simulink library "CampusEnergyModeling"  (Simulink 8.1)
settings: Solver=ode45  StartTime=0.0  StopTime=10.0  RelTol=1e-3
undefined symbols (not defined in the file): a, b, c, j, look_Pin, look_Pout, magnitude
libraries: powerlib x6, simulink x3
(part 1 of 2)
settings Model: Creator=sfrank1  LastModifiedBy=sfrank1

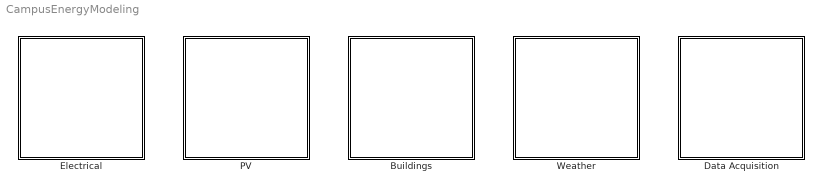
== system CampusEnergyModeling ==
  Buildings : Subsystem  Tag=Weather  Description=Contains blocks for acquiring and manipulating weather data.
      mask Display: disp('Buildings')
  Data Acquisition : Subsystem  Tag=Weather  Description=Contains blocks for acquiring and manipulating weather data.
      mask Display: disp('Data\nAcquisition')
  Electrical : Subsystem  Tag=Weather  Description=Contains blocks for acquiring and manipulating weather data.
      mask Display: disp('Electrical')
  PV : Subsystem  Tag=Weather  Description=Contains blocks for acquiring and manipulating weather data.
      mask Display: disp('PV')
  Weather : Subsystem  Tag=Weather  Description=Contains blocks for acquiring and manipulating weather data.
      mask Display: disp('Weather')

== system CampusEnergyModeling/Buildings ==
  EnergyPlus : M-S-Function  FunctionName=mlep_sfun  Parameters=work_dir, rel_path, fname, weather_profile, time_step, nout, timeout, eplus_path, bcvtb_dir, port, host  mask(EnergyPlus Cosimulation){work_dir=, rel_path=on, fname=idf_file, weather_profile=USA_IL_Chicago-OHare.Intl.AP.725300_TMY3, time_step=900, nout=2, timeout=10, mlep_defaults=on, eplus_path=, bcvtb_dir=, port=0, host=}
      mask prompts: work_dir "MLE+ working directory (empty = current directory)"; rel_path "Relative path"; fname "IDF file name"; weather_profile "EnergyPlus weather profile"; time_step "Time step (s)"; nout "Number of real outputs"; timeout "Communication timeout (s)"; mlep_defaults "Use default MLE+ settings"; eplus_path "EnergyPlus executable path (empty = default)"; bcvtb_dir "BCVTB directory (empty = default)"; port "Socket port (0 = auto)"; host "Socket host (empty = localhost)"
      mask help: This block implements cosimulation with EnergyPlus by allowing Simulink to exchange input and output data with it. Currently, EnergyPlus only supports real data.
      mask Help:
      | Simulate a building model using EnergyPlus
      | 
      | <h2>Description</h2>
      | This block implements <a href="http://apps1.eere.energy.gov/buildings/energyplus/">EnergyPlus</a> cosimulation by allowing Simulink to exchange input and output data with EnergyPlus at each time step.
      | 
      | When a simulation starts, this block starts EnergyPlus in parallel. During simulation, EnergyPlus exchanges data with Simulink using the <a href="http://simulationresearch.lbl.gov/bcvtb">Building Controls Virtual Test Bed</a> (BCVTB) interface via <a href="http://mlab.seas.upenn.edu/mlep/">MLE+</a>.
      | 
      | Detailed information about the interface is available in the MLE+ manual.
      | 
      | <h2>Requirements</h2>
      | Requires <a href="http://apps1.eere.energy.gov/buildings/energyplus/">EnergyPlus</a> and <a href="http://mlab.seas.upenn.edu/mlep/">MLE+</a>. In addition, requires a properly configured EnergyPlus model file (IDF) and BCVTB configuration file; see Comments.
      | 
      | <h2>Input</h2>
      | Block input <b>input</b> is a real-valued vector of EnergyPlus inputs corresponding to the inputs listed in the BCVTB config file <code>variables.cfg</code> (in order).
      | 
      | <h2>Output</h2>
      | The block outputs are, in order:
      | <dl>
      |   <dt><b>flag</b></dt><dd>Status flag for EnergyPlus: 0 if OK, non-zero for error</dd>
      |   <dt><b>time</b></dt><dd>Current simulation time of EnergyPlus (s)</dd>
      |   <dt><b>output</b></dt><dd>Real-valued vector of EnergyPlus outputs corresponding to the outputs listed in the BCVTB config file <code>variables.cfg</code> (in order).</dd>
      | </dl>
      | 
      | <h2>Parameters</h2>
      | The block mask provides inputs for all required MLE+ configuration parameters. The mask includes two tabs. The <i>Model</i> tab provides information about the EnergyPlus model to run, and the <i>MLE+</i> provides inputs for MLE+ settings.
      | 
      | String inputs in the block mask, such as paths and file names, are not evaluated prior to passing to MLE+. Therefore, MATLAB expressions which evaluate to strings (for example, <code>[pwd '/somedir']</code>) may not be passed directly. Instead, use an initialization script to evaluate these expressions and store the evaluated strings in the block mask prior to running the simulation.
      | 
      | <h3>Model Tab</h3>
      | The <i>Model</i> tab provides inputs for the following parameters:
      | <dl>
      |   <dt><b>MLE+ working directory</b></dt>
      |     <dd>The MLE+ and EnergyPlus working directory. <i>EnergyPlus will read from and write to this directory.</i></dd>
      |   <dt><b>Relative path</b></dt>
      |     <dd>Check this box if <b>MLE+ working directory</b> is specified relative to the current MATLAB working directory. <i>Otherwise, the block will treat <b>MLE+ working directory</b> as an absolute path.</i></dd>
      |   <dt><b>IDF file name</b></dt>
      |     <dd>The EnergyPlus model file (IDF), with or without the <code>.idf</code> extension. <i>This file must be included in the <b>MLE+ working directory</b>. Do not specify an absolute path for this file!</i></dd>
      |   <dt><b>EnergyPlus weather profile</b></dt>
      |     <dd>The EnergyPlus weather file (EPW), with or without the <code>.epw</code> extension. <i>A matching weather file must be included in your EnergyPlus installation's <code>WeatherData</code> directory.</i></dd>
      |   <dt><b>Time Step</b></dt>
      |     <dd>The EnergyPlus time step (s). <i>This need not be the same as the Simulink time step.</i></dd>
      |   <dt><b>Number of Real Outputs</b></dt>
      |     <dd>The number of real outputs from EnergyPlus. <i>This number must match the number of output variables in <code>variables.cfg</code>.</i></dd>
      | </dl>
      | 
      | <h3>MLE+ Tab</h3>
      | The <i>MLE+</i> tab provides inputs for the following parameters:
      | <dl>
      |   <dt><b>Communication timeout</b></dt>
      |     <dd>Time delay (s) before communication between MLE+ and EnergyPlus times out.</dd>
      |   <dt><b>Use default MLE+ settings</b></dt>
      |     <dd>Uncheck this box to gain access to the remaining settings in the <i>MLE+</i> tab.</dd>
      |   <dt><b>EnergyPlus executable path</b></dt>
      |     <dd>The full path to the EnergyPlus executable (e.g. <code>C:\EnergyPlusV8-1-0\RunEPlus.bat</code>); leave blank to use default MLE+ setting.</dd>
      |   <dt><b>BCVTB directory</b></dt>
      |     <dd>The full path to the directory where the BCVTB library resides; leave blank to use default MLE+ setting.</dd>
      |   <dt><b>Socket port</b></dt>
      |     <dd>The port to use for communication with EnergyPlus; enter <code>0</code> to allow MLE+ to automatically select a port.</dd>
      |   <dt><b>Socket host</b></dt>
      |     <dd>The IP address of the host machine where EnergyPlus runs; leave blank to use localhost (the local computer).</dd>
      | </dl>
      | 
      | <h2>Comments</h2>
      | <ol>
      |   <li>For fixed time step simulation in Simulink, the EnergyPlus time step must be an exact multiple of the Simulink time step.</li>
      |   <li>Summary of requirements for EnergyPlus model file (<code>*.idf</code>):
      |     <ol type="a">
      | 	  <li>The EnergyPlus time step specified in the file must match the value specified in the block mask.</li>
      | 	  <li>The start date and time in EnergyPlus must correspond to the start time of the Simulink simulation (usually <i>t</i> = 0 s).</li>
      | 	  <li>The <i>ExternalInterface</i> object must be defined and assigned the name  <code>PtolemyServer</code>.</li>
      | 	  <li>The file must include <i>ExternalInterface</i> definitions all inputs specified in the BCVTB config file, and the names must match.</li>
      | 	  <li>The file must include <i>Output</i> definitions all outputs specified in the BCVTB config file, and the names must match.</li>
      | 	</ol>
      |   </li>
      |   <li>Summary of requirements for BCVTB config file (<code>variables.cfg</code>):
      |     <ol type="a">
      | 	  <li>The file be located in the MLE+ working directory specified in the block mask.</li>
      | 	  <li>Number of output variables must match the value specified in the block mask.</li>
      | 	  <li>Order of input variables must match the order of elements in the input vector in Simulink.</li>
      | 	  <li>Order of output variables must match the order of elements in the output vector in Simulink.</li>
      | 	</ol>
      |   <li>For more details regarding the implementation of MLE+, the meaning of the parameters, and creating the BCVTB configuration file, see the MLE+ <a href="http://mlab.seas.upenn.edu/mlep/">documentation</a>.</li>
      | </ol>
      | 
      | <h2>References</h2>
      | <ol>
      |   <li>W. Bernal, M. Behl, T. X. Nghiem, and R. Mangharam, "MLE+: A Tool for Integrated Design and Deployment of Energy Efficient Building Controls," 4th ACM Workshop On Embedded Sensing Systems For Energy-Efficiency In Buildings, (BuildSys '12), Toronto, Canada, 2012. Available: <a href="http://repository.upenn.edu/mlab_papers/51/">http://repository.upenn.edu/mlab_papers/51/</a></li>
      | </ol>
      mask Callback mlep_defaults: EnergyPlus_cb(gcb, 'mlep_config');
      mask Display:
      | image(imread('building.png'))
      | disp('EnergyPlus\nCosimulation');
      | 
      | % Inputs
      | port_label('input', 1, 'input');
      | 
      | % Outputs
      | port_label('output', 1, 'flag');
      | port_label('output', 2, 'time');
      | port_label('output', 3, 'output');

== system CampusEnergyModeling/Data Acquisition ==

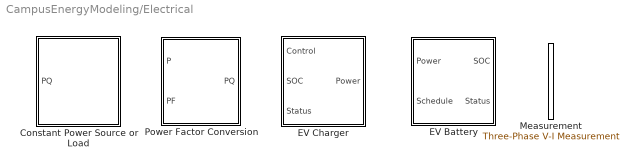
== system CampusEnergyModeling/Electrical ==
  Constant Power Source or Load : Subsystem  mask(Constant Power Source/Load){Conven=source, PNom=5000, QNom=2000, VNom=480, fNom=60, VLow=0.7}
      mask prompts: Conven "Electrical convention"; PNom "Nominal three-phase real power (W)"; QNom "Nominal three-phase reactive power (VAR)"; VNom "Nominal line-to-line voltage (VRMS)"; fNom "Nominal frequency (Hz)"; VLow "Lower voltage limit (pu)"
      mask help: Implements a controllable three-phase, constant power source or load, where VI* = P + jQ (in per-unit).
      mask init:
      | % Call initialization to calculate block variables
      | InputGain = ...
      |     ConstantPowerSourceLoad_cb(gcb, 'init', ...
      |     Conven, PNom, QNom, VNom, fNom, VLow);
      mask Help:
      | Supply or consume constant three-phase power
      | 
      | <h2>Description</h2>
      | This block implements a controllable three-phase, constant power source or load in SimPowerSystems (phasor mode). The load characteristic is given by
      | <blockquote>
      |   <i>P</i> + <i>jQ</i> = sqrt(3) · <i>VI</i><sup>*</sup>,
      | </blockquote>
      | in which
      | <blockquote>
      |   <i>V</i> = Positive sequence line-to-line voltage (V)<br/>
      |   <i>I</i> = Positive sequence phase current (A)<br/>
      |   <i>P</i> = Positive sequence real power (from PQ input)<br/>
      |   <i>Q</i> = Positive sequence reactive power (from PQ input)
      | </blockquote>
      | 
      | The block supplies <i>P</i> + <i>jQ</i> if the source convention is specified and consumes <i>P</i> + <i>jQ</i> if the load convention is specified.
      | 
      | <h2>Requirements</h2>
      | Requires SimPowerSystems.
      | 
      | <h2>Input</h2>
      | Input <b>PQ</b> is a two dimensional vector [<i>P</i>, <i>Q</i>] specifying the real and reactive power consumption (for a load) or generation (for a source).
      | 
      | <h2>Physical Ports</h2>
      | <p>The block has a three-phase, four-wire physical representation in SimPowerSystems. The physical ports are:
      | <dl>
      |   <dt><b>A</b></dt><dd>Phase A electrical connection</dd>
      |   <dt><b>B</b></dt><dd>Phase B electrical connection</dd>
      |   <dt><b>C</b></dt><dd>Phase C electrical connection</dd>
      |   <dt><b>N</b></dt><dd>Neutral electrical connection</dd>
      | </dl>
      | </p>
      | 
      | <h2>Parameters</h2>
      | <dl>
      |   <dt><b>Electrical convention</b></dt>
      |     <dd>Specifies whether the block is a source or a load</dd>
      |   <dt><b>Nominal three-phase real power</b></dt>
      |     <dd>The nominal real power production (consumption) for the source (load), in W</dd>
      |   <dt><b>Nominal three-phase reactive power</b></dt>
      |     <dd>The nominal reactive power production (consumption) for the source (load), in W</dd>
      |   <dt><b>Nominal line-to-line voltage</b></dt>
      |     <dd>The nominal line-to-line voltage, in V</dd>
      |   <dt><b>Nominal frequency</b></dt>
      |     <dd>The nominal frequency of the device, in Hz</dd>
      |   <dt><b>Lower voltage limit</b></dt>
      |     <dd>The voltage below which the block converts to a constant current device; see Comments</dd>
      | </dl>
      | 
      | <h2>Comments</h2>
      | <ol>
      |   <li>This block is compatible with SimPowerSystems' <b>phasor simulation mode only.</b></li>
      |   <li>The nominal input fields in the mask are used to initialize the block parameters. If the nominal values are close to the actual values during simulation, then the block will converge more rapidly.</li>
      |   <li>If the positive sequence voltage falls below the per-unit lower voltage limit (on the base specified by the nominal line-to-line voltage), then the block will behave as a constant current source rather than a constant power source, with the current magnitude capped at the level required to supply full power at the lower voltage limit. This feature avoids current runaway that would otherwise occur during voltage collapes. By default, the lower voltage limit is <i>V</i> = 0.7 pu.
      | </ol>
      mask TypeOptions Conven: source | load
  EV Battery : Subsystem  mask(Electric Vehicle Battery){capacity=24000, initSOC=0.3}
      mask prompts: capacity "Battery capacity (Wh)"; initSOC "Initial state of charge (fraction)"
      mask help: Implements an idealized (lossless) model for an electric vehicle (EV) battery.
      mask Help:
      | Models a lossless electric vehicle battery
      | 
      | <h2>Description</h2>
      | This block models an idealized (lossless) electric vehicle (EV) battery. The battery is modeled using a simple integrator on the input power, capped at 100% state of charge (SOC). Battery SOC resets to a specified initial value whenever the EV reconnects to the charging station (whenever the <b>Schedule</b> input transitions from 0 to 1).
      | 
      | <h2>Input</h2>
      | <dl>
      |   <dt><b>Power</b></dt>
      |     <dd>Battery charging power (W)</dd>
      |   <dt><b>Schedule</b></dt>
      |     <dd>EV schedule:
      |         <ul>
      |           <li>1 (or any other positive number) if the EV is connected to the charging station,</li>
      |           <li>0 otherwise.</li>
      |         </ul>
      |     </dd>
      |     </dl>
      | </dl>
      | 
      | <h2>Output</h2>
      | <dl>
      |   <dt><b>SOC</b></dt>
      |     <dd>EV battery current state of charge (fraction); compatible with the <b>SOC</b> input of the <i>EV Charger</i> block</dd>
      |   <dt><b>Status</b></dt><dd>EV status:
      |     <ul>
      |       <li>&minus;1 for not present,</li>
      |       <li>0 for present and accepting charge,</li>
      |       <li>1 for present but battery full;</li>
      |     </ul>
      |     compatible with the <b>Status</b> input of the <i>EV Charger</i> block</dd>
      | </dl>
      | 
      | <h2>Parameters</h2>
      | <dl>
      |   <dt><b>Battery capacity</b></dt>
      |     <dd>EV battery storage capacity (Wh)</dd>
      |   <dt><b>Initial state of charge</b></dt>
      |     <dd>Initial battery SOC when the battery first reconnects to the charging station (fraction)</dd>
      | </dl>
  EV Charger : Subsystem  mask(Electric Vehicle Charging Station){rating=6240, capacity=24000, maxresponse=1000, ramp=1000}
      mask prompts: rating "Charger rating (W)"; capacity "Connected EV battery capacity (Wh)"; maxresponse "Desired +/- regulatory response capability (W)"; ramp "Maximum ramp rate (W/s)"
      mask help: Implements a simple model for an electric vehicle charging station. Accepts connections for the EV state of charge and status as well as an external control signal requesting a regulatory deviation from the current charging setpoint. Outputs a charging power.
      mask Help:
      | Models an electric vehicle charging station
      | 
      | <h2>Description</h2>
      | This block models an idealized electric vehicle (EV) charging station. It is an approximation of how actual EV charging stations operate (to be updated in a later release of the library). The charger uses a preset charging power profile based on the EV battery state of charge (SOC). As the SOC approaches 100%, the charger tapers the charge rate to zero. In addition, the charger monitors the connection status of the EV and sets charging power to zero if the EV is disconnected or has a full battery.
      | 
      | The block has a <b>Control</b> signal which requests regulatory control of the EV charging load as a deviation from the current charging setpoint. This allows the EV charger to participate in demand response or regulation of distributed generation (such as smoothing output from a photovoltaic array). The charger attempts to maintain the active response capability specified in the block mask by operating at less than maximum charging capacity. It can then respond to the control signal within its present charging limits. See Comments for details.
      | 
      | <h2>Input</h2>
      | <dl>
      |   <dt><b>Control</b></dt>
      |     <dd>Signal requesting regulatory control of charging power (&plusmn; deviation from charging setpoint) (W)</dd>
      |   <dt><b>SOC</b></dt>
      |     <dd>EV battery current state of charge (fraction); compatible with the <b>SOC</b> output of the <i>EV Battery</i> block</dd>
      |   <dt><b>Status</b></dt>
      |     <dd>EV status:
      |     <ul>
      |       <li>&minus;1 for not present,</li>
      |       <li>0 for present and accepting charge,</li>
      |       <li>1 for present but battery full;</li>
      |     </ul>
      |     compatible with the <b>Status</b> output of the <i>EV Battery</i> block</dd>
      | </dl>
      | 
      | <h2>Output</h2>
      | Output <b>Power</b> is the charger power output (W).
      | 
      | <h2>Parameters</h2>
      | <dl>
      |   <dt><b>Charger rating</b></dt>
      |     <dd>The charger maximum power rating (W)</dd>
      |   <dt><b>Connected EV battery capacity</b></dt>
      |     <dd>The total energy storage capacity of the connected EV battery (Wh)</dd>
      |   <dt><b>Desired +/- regulatory response capability</b></dt>
      |     <dd>The target control response capability (W) for the charger</dd>
      |   <dt><b>Maximum ramp rate</b></dt>
      |     <dd>Maximum charging ramp rate (&plusmn; rate of change in charging power) (W/s)</dd>
      | </dl>
      | 
      | <h2>Comments</h2>
      | Internally, the block sets a maximum charge rate based on the EV battery capacity and current SOC. The charging setpoint is the maximum rate less any requested regulatory response capability. The actual charging power is equal to this setpoint plus the effect of the control signal.
      | 
      | The ability of the charger to respond to the requested control action is limited by four factors:
      | <ol>
      |   <li>The output power cannot exceed the specified charger power rating.</li>
      |   <li>The output power cannot exceed the maximum charge rate defined by the battery charging profile.</li>
      |   <li>The output power cannot be less than zero. (The battery cannot be discharged to the grid.)</li>
      |   <li>The output power cannot change at a rate greater than the specified maximum ramp rate.</li>
      | </ol>
      | 
      | <i>Example:</i> If, given the current battery SOC, the charging profile for the EV battery specifies 5000 W and the requested regulatory response capability is &plusmn;1000 W, then the EV charger will charge at a setpoint of 4000 W &plusmn; the requested control action, within the limits of the charger. If the requested control action is &minus;500 W, then the EV charger will reduce output to 4000 &minus; 500 = 3500 W.
  Measurement : powerlib/Measurements/Three-Phase V-I Measurement  VoltageMeasurement=phase-to-ground  SetLabelV=on  LabelV=Vabc_1  Vpu=off  VpuLL=off  CurrentMeasurement=yes  SetLabelI=on  LabelI=Iabc_1  Ipu=off  Pbase=1e6  Vbase=25e3  OutputType=Complex  PhasorSimulation=on  PSBequivalent=0
  Power Factor Conversion : Subsystem  mask(Power Factor Conversion){pfType=Lagging}
      mask prompts: pfType "Type of power factor"
      mask help: Converts a real input power and power factor to a vector of real and reactive power.
      mask init:
      | % Set multiplier for Q based on load type
      | if pfType == 1
      |     % Leading
      |     leadlag = -1;
      | else
      |     % Lagging
      |     leadlag = 1;
      | end
      mask Help:
      | Convert from real power and power factor to real and reactive power
      | 
      | <h2>Description</h2>
      | 
      | Given a real input power and power factor, this block computes a vector of real and reactive power (compatible with the <i>Constant Power Source/Load</i> block). Reactive power <i>Q</i> in output vector [<i>P</i>, <i>Q</i>] is given by
      | <blockquote>
      |   <i>Q</i> = &plusmn;<i>P</i> · sqrt( 1 + 1 / PF&sup2; ),
      | </blockquote>
      | with the sign determined by whether the power factor is assumed to be lagging (+) or leading (&minus;) (selectable in the block mask).
      | 
      | <h2>Input</h2>
      | Input <b>P</b> is the real power and input <b>PF</b> is the power factor.
      | 
      | <h2>Output</h2>
      | Output <b>PQ</b> is a two dimensional vector [<i>P</i>, <i>Q</i>] of the computed real and reactive power.
      | 
      | <h2>Parameters</h2>
      | The <b>type of power factor</b> parameter is a drop-down list which specifies whether the power factor is leading or lagging.
      mask TypeOptions pfType: Leading | Lagging

== system CampusEnergyModeling/PV ==
  Generic Inverter : Subsystem  mask(Generic Inverter){model_type=Fixed Efficiency, fixed_eff=0.95, alpha=1, beta=0.01, gamma=0.001, lookup_pair=Input Power + Output Power, lookup_in=[0, 10, 25, 50, 75, 100], lookup_out=[0, 9, 24, 49, 73, 97], lookup_eff=[0.10, 0.80, 0.87, 0.93, 0.90, 0.88], standby=0}
      mask prompts: model_type "Inverter model"; fixed_eff "Efficiency"; alpha "Constant loss coefficient (W)"; beta "Linear loss coefficient (W/W)"; gamma "Quadratic loss coefficient (W/W²)"; lookup_pair "Specify..."; lookup_in "Input power (W)"; lookup_out "Output power (W)"; lookup_eff "Efficiency"; standby "Standby Loss (W)"
      mask help:
      | Implements the efficiency characteristic for a generic PV inverter using one of three models:
      | - Fixed efficiency
      | - Quadratic loss model
      | - Lookup table
      |
      | See the help for details for each of these models.
      mask init:
      | % Call initialization to calculate block variables
      | [a, b, c, look_Pin, look_Pout] = ...
      |     GenericInverter_cb(gcb, 'init', model_type, ...
      | 	fixed_eff, alpha, beta, gamma, ...
      |     lookup_pair, lookup_in, lookup_out, lookup_eff);
      mask Help:
      | Simulate the efficiency characteristic of a generic PV inverter
      | 
      | <h2>Description</h2>
      | The block simulates the efficiency characteristic of a generic photovoltaic (PV) inverter using one of three models:
      | <ul>
      |   <li>Fixed efficiency</li>
      |   <li>Quadratic loss model</li>
      |   <li>Lookup table</li>
      | </ul>
      | 
      | <h3>Fixed Efficiency Model</h3>
      | Under the fixed efficiency model, the inverter power output is a fixed fraction of the input: <i>P<sub>out</sub></i> = <i>&eta;</i><i>P<sub>in</sub></i>. Efficiency <i>&eta;</i> is a mask parameter.
      | 
      | <h3>Quadratic Loss Model</h3>
      | Under the quadratic loss model, inverter losses are a quadratic function of the inverter input power. The power relationship is <i>P<sub>out</sub></i> = <i>P<sub>in</sub></i> - ( <i>&alpha;</i> + <i>&beta;</i><i>P<sub>in</sub></i> + <i>&gamma;</i><i>P<sub>in</sub></i>²). <i>&alpha;</i>, <i>&beta;</i>, and <i>&gamma;</i> are the constant, linear, and quadratic loss coefficients, respectively, and are mask parameters.
      | 
      | <h3>Lookup Table</h3>
      | Inverter output power is computed as a function of the input power using interpolation from a preset lookup table.
      | 
      | <h2>Input</h2>
      | Block input <b>Pin</b> is the inverter input power.
      | 
      | <h2>Output</h2>
      | Block output <b>Pout</b> is the inverter output power.
      | 
      | <h2>Parameters</h2>
      | <b>Standby loss</b> (W) specifies the inverter power consumption when the array is dark. The remaining parameters available in the block mask depend on which <b>inverter model</b> is selected in the mask dialog.
      | 
      | <h3>Fixed Efficiency Model</h3>
      | Specify the fixed inverter <b>efficiency</b> <i>&eta;</i> as a fraction.
      | 
      | <h3>Quadratic Loss Model</h3>
      | Specify <i>&alpha;</i>, <i>&beta;</i>, and <i>&gamma;</i> in the inverter loss equation:
      | <dl>
      |   <dt><b>Constant loss coefficient</b></dt><dd>Specify the constant inverter loss <i>&alpha;</i> (W).</dd>
      |   <dt><b>Linear loss coefficient</b></dt><dd>Specify the linear inverter loss coefficient <i>&beta;</i> (W/W).</dd>
      |   <dt><b>Quadratic loss coefficient</b></dt><dd>Specify the quadratic inverter loss coefficient <i>&gamma;</i> W/W²).</dd>
      | </dl>
      | 
      | <h3>Lookup Table</h3>
      | Specify two of the following three vectors: <b>input power</b>, <b>output power</b>, and <b>efficiency</b>. Vector dimensions must match and efficiencies must be entered as fractions. The block automatically calculates the appropriate input-output power characteristic from the inputs provided according to the relationship <i>&eta;</i> = <i>P<sub>out</sub></i> / <i>P<sub>in</sub></i>.
      | 
      | <h2>Comments</h2>
      | <ol>
      |   <li>When the inverter input power drops too low to sustain a positive power output, the inverter drops into standby automatically, consuming the specified standby loss.</li>
      |   <li><i>Caution:</i> If using the lookup table model, do not include zeros in the efficiency vector. Otherwise, a divide by zero error may result.</li>
      | </ol>
      | 
      | <h2>References</h2>
      | For discussion of the quadratic inverter loss model, see section 3.4.4 of:
      | <ol>
      |   <li>S. Frank, "Optimal Design of Mixed AC-DC Distribution Systems for Commercial Buildings," Dissertation, Colorado School of Mines, Golden, CO, 2013. Available: <a href="http://gradworks.umi.com/3558161.pdf">http://gradworks.umi.com/3558161.pdf</a></li>
      | </ol>
      mask TypeOptions model_type: Fixed Efficiency | Quadratic | Lookup Table
      mask Callback model_type:
      | % Dynamic mask callback
      | GenericInverter_cb(gcb, 'model_type')
      mask TypeOptions lookup_pair: Input Power + Output Power | Input Power + Efficiency | Output Power + Efficiency
      mask Callback lookup_pair:
      | % Dynamic mask callback
      | GenericInverter_cb(gcb, 'lookup_pair')
  PV Smoothing : TransferFcn  Denominator=[tau 1]  mask(Photovoltaic Array Smoothing){sel=Array Size and Power Density, tc=15, area=33000, size=1e6, density=150, coverage=0.2}
      mask prompts: sel "Specify..."; tc "Time constant (s)"; area "Array area (m²)"; size "Array size (W)"; density "Panel nominal power density (W/m²)"; coverage "Panel ground coverage ratio (fraction)"
      mask help: Implements a low pass filter to model the smoothing effect of a utility-scale PV array.
      mask init:
      | % Call initialization to calculate block variables
      | tau = PVSmoothing_cb(gcb, 'init', ...
      |     sel, tc, area, size, density, coverage);
      mask Help:
      | Model the smoothing effect of a utility-scale PV array
      | 
      | <h2>Description</h2>
      | This block implements a low pass filter to model the smoothing effect of a utility-scale PV array per the empirical model presented in Marcos et al. (2011) (see References). The smoothing is done by a unity-gain low pass filter with transfer function
      | <blockquote>
      |   Output / Input = 1 / (<i>&tau;</i><i>s</i> + 1),
      | </blockquote>
      | in which time constant <i>&tau;</i> may either be defined directly or estimated from the array area. The empirical formula of Marcos et al. estimates <i>&tau;</i> as
      | <blockquote>
      |   <i>&tau;</i> = sqrt(<i>A</i>) / (2·&pi;·0.020)
      | </blockquote>
      | in which <i>A</i> is the physical array area in hectares (1 Ha = 10000 m&sup2;). Array area <i>A</i> may be specified directly or calculated from the array size, panel power density, and ground coverage ratio (defined as the fraction of ground area occupied by the actual PV panels).
      | 
      | <h2>Input</h2>
      | Block input <b>Pin</b> is the unsmoothed PV array power.
      | 
      | <h2>Output</h2>
      | Block output <b>Pout</b> is the smoothed PV array power.
      | 
      | <h2>Parameters</h2>
      | In the mask dialog, the user elects to specify the time constant, the array area, or the array size and power density.
      | 
      | <h3>Time Constant</h3>
      | Specify the <b>time constant</b> (s) for the low pass filter directly.
      | 
      | <h3>Array Area</h3>
      | Specify the <b>array area</b> (m&sup2;) and compute the time constant from the equation of Marcos et al. (2011).
      | 
      | <h3>Time Constant</h3>
      | Specify the <b>array size</b> (W), <b>nominal power density</b> (W/m&sup2;), and <b>ground coverage ratio</b> (fraction). From this, the block computes the approximate array area and the time constant from the equation of Marcos et al. (2011).
      | 
      | <h2>Comments</h2>
      | <ol>
      |   <li>This block includes a continuous time low pass filter. Therefore, the block may not be used with a discrete solver. Also, use caution when attempting to use this block within models with fixed time larger than the smoothing time constant; the Simulink solver may generate an error.</li>
      | </ol>
      | 
      | <h2>References</h2>
      | <ol>
      |   <li>J. Marcos et al., "From irradiance to output power fluctuations: the PV plant as a low pass filter", <i>Progress In Photovoltaics: Research And Applications</i>, 2011, 19, 505-510.</li>
      | </ol>
      mask TypeOptions sel: Time Constant | Array Area | Array Size and Power Density
      mask Callback sel: PVSmoothing_cb(gcb, 'dynamic_mask')
      mask Display: plot([1 2 3],[1 1 0])
  PVWatts Cosimulation : M-S-Function  FunctionName=pvwatts_sfun  Parameters=lat, lon, start_time, tz, time_step, system_size, derate, azimuth, tilt, track_mode, rotlim, t_ref, t_noct, gamma, i_ref, poa_cutin, init_tcell, init_poa, output_dc, output_celltemp, output_poa  mask(PVWatts Cosimulation){lat=39.74, lon=-105.18, start_time=2012-01-01 00:00:00, tz=-6, time_step=600, system_size=1000, derate=0.95, azimuth=180, tilt=39.74, use_lat_tilt=on, track_mode=Fixed, rotlim=45, use_cell_data=off, t_ref=25, t_noct=45, gamma=-0.5, i_ref=1000, poa_cutin=0, init_tcell=25, init_poa=0, output_dc=on, output_celltemp=on, output_poa=on}
      mask prompts: lat "Latitude"; lon "Longitude"; start_time "Initial date/time (yyyy-mm-dd HH:MM:SS)"; tz "Time zone (offset from UTC)"; time_step "Time step (s)"; system_size "Array nameplate capacity (W)"; derate "System derate factor (0-1)"; azimuth "Azimuth angle (N = 0°, E = 90°, S = 180°, W = 270°)"; tilt "Tilt angle"; use_lat_tilt "Use latitude tilt"; track_mode "Tracking mode"; rotlim "Tracker rotation limit (+/-)"; use_cell_data "Customize photovoltaic cell data"; t_ref "Reference cell temperature (°C)"; t_noct "Nominal operating cell temperature (°C)"; gamma "Maximum power temperature coefficient (%/°C)"; i_ref "Irradiance condition for cell rating (W/m²)"; poa_cutin "Minimum irradiance for operation (W/m²)"; init_tcell "Initial cell temperature (°C)"; init_poa "Initial plane of array irradiance (W/m²)"; output_dc "Output DC power (W)"; output_celltemp "Output cell temperature (°C)"; output_poa "Output plane of array irradiance (W/m²)"
      mask help:
      | This block implements cosimulation of a photovoltaic (PV) array using the PVWatts module of the SAM Simulation Code (SSC) SDK. Data entry is organized in four tabs:
      | 1. Time and Location: where the array is located and when the simulation occurs.
      | 2. Array: PV array nameplate rating and physical characteristics.
      | 3. Cell: Customized model parameters for the PV cells (optional).
      | 4. Simulation: Initial conditions and simulation options.
      |
      | See the block help for more information.
      mask init:
      | PVWatts_cb(gcb, 'redraw_mask');
      mask Help:
      | Simulate a photovoltaic array using PVWatts
      | 
      | <h2>Description</h2>
      | This block implements cosimulation of a photovoltaic (PV) array using the PVWatts (<code>pvwattsfunc</code>) module of the SAM Simulation Core (SSC) SDK. The cosimulation runs in SSC at the time step specified in the <i>Time and Location</i> parameter tab (which need not be identical to the Simulink time step).
      | 
      | Detailed documentation for the SSC SDK is available for download from the <a href="https://sam.nrel.gov/content/sam-simulation-core-sdk">SAM website<a/>; see References.
      | 
      | <h2>Requirements</h2>
      | Requires <a href="https://sam.nrel.gov/content/sam-simulation-core-sdk">SSC</a>.
      | 
      | <h2>Input</h2>
      | The block inputs accept weather data synced to the simulation time stamp:
      | <dl>
      |   <dt><b>Beam</b></dt><dd>Beam irradiance (W/m&sup2;)—Also known as "direct normal irradiance"</dd>
      |   <dt><b>Diffuse</b></dt><dd>Diffuse irradiance (W/m&sup2;)—Also known as "diffuse horizontal irradiance"</dd>
      |   <dt><b>Temp</b></dt><dd>Ambient temperature (&deg;C)</dd>
      |   <dt><b>Wind</b></dt><dd>Wind speed (m/s)</dd>
      | </dl>
      | 
      | <h2>Output</h2>
      | The block outputs are, in order:
      | <dl>
      |   <dt><b>DC Power</b></dt><dd>Array DC output power (W)</dd>
      |   <dt><b>Cell Temp</b></dt><dd>Array PV cell temperature (&deg;C)</dd>
      |   <dt><b>POA Irradiance</b></dt><dd>Plane of array incident irradiance (W/m&sup2;)</dd>
      | </dl>
      | 
      | Each output may be individually enabled or disabled on the <i>Simulation</i> tab. Enabling or disabling outputs will change the number of output ports on the block, possibly disrupting existing signal connections in Simulink.
      | 
      | <h2>Parameters</h2>
      | The block mask provides inputs for most (although not all) of the PV array model parameters available for PVWatts in SSC. The four input tabs in the block mask are
      | <ol>
      |   <li><i>Time and Location:</i> Specify where the array is located and when the simulation occurs. Includes fields for array <b>latitude</b> and <b>longitude</b>, the <b>initial date and time</b> (corresponding to simulation time <i>t</i> = 0), <b>time zone</b>, and PVWatts simulation <b>time step.</b></li>
      |   <li><i>Array:</i> Specify the PV array <b>nameplate capacity</b>, <b>derate factor</b>, and physical characteristics (<b>azimuth angle</b>, <b>tilt angle</b>, and <b>tracking mode</b>).</li>
      |   <li><i>Cell:</i> Allows customization of the photovoltaic cell data—<b>reference cell temperature</b>, <b>nominal operating cell temperature</b>, <b>maximum power temprature coefficient</b>, <b>irradiance condition</b> for cell rating, and <b>minimum irradiance</b> for cell operation.</li>
      |   <li><i>Simulation:</i> Specify the array initial conditions (<b>cell temperature</b> and <b>plane of array irradiance)</b> and select the desired block outputs.</li>
      | </ol>
      | 
      | For a detailed description of these parameters, see the SSC SDK documentation.
      | 
      | <h2>Comments</h2>
      | <ol>
      |   <li>The block is designed to model the DC operation of a PV array only. Therefore, no inverter efficiency mask parameter or AC power output are provided. To model inverter losses, apply an external inverter model to the DC power output, such as the Generic Inverter model available in the Campus Energy Modeling Simulink library.</li>
      |   <li><i>Caution:</i> Checking <b>Use latitude tilt</b> in the <i>Array</i> tab will discard the existing tilt angle and replace it with the absolute value of the latitude.</li>
      |   <li><i>Caution:</i> Unchecking <b>Customize photovoltaic cell data</b> in the <i>Cell</i> tab will discard any existing customizations in the PV cell data fields and replace them with default values.</li>
      |   <li>Additional description for the SSC module input and output variables may be obtained using the SSCdev application distributed with SSC SDK; see the SSC SDK documentation for usage instructions.</li>
      | </ol>
      | 
      | <h2>References</h2>
      | <ol>
      |   <li>National Renewable Energy Laboratory, "SAM Simulation Core SDK." Available: <a href="https://sam.nrel.gov/content/sam-simulation-core-sdk">https://sam.nrel.gov/content/sam-simulation-core-sdk</a></li>
      | </ol>
      mask Callback lat: PVWatts_cb(gcb, 'use_lat_tilt');
      mask Callback use_lat_tilt: PVWatts_cb(gcb, 'use_lat_tilt');
      mask TypeOptions track_mode: Fixed | 1-Axis | 2-Axis | Azimuth Axis
      mask Callback track_mode: PVWatts_cb(gcb, 'track_mode');
      mask Callback use_cell_data: PVWatts_cb(gcb, 'use_cell_data');
      mask Display:
      | % This mask display is automatically generated by PVWatts_cb()
      | image('pvwatts_light.png')
      | disp('PVWatts\nCosimulation')
      | 
      | % Label input ports
      | port_label('input', 1, 'Beam'); % Beam irradiance (W/m^2)
      | port_label('input', 2, 'Diffuse'); % Diffuse irradiance (W/m^2)
      | port_label('input', 3, 'Temp'); % Ambient temperature (deg C)
      | port_label('input', 4, 'Wind'); % Wind speed (m/s)
      | 
      | % Label output ports
      | port_label('output', 1, 'DC Power'); % DC output power (W)
      | port_label('output', 2, 'Cell Temp'); % Cell temperature (deg C)
      | port_label('output', 3, 'POA Irradiance'); % % Point of array irradiance

== system CampusEnergyModeling/Weather ==
  Weather Data : Subsystem  mask(Weather Data From File){fname=TMY3.mat, initbus=off}
      mask prompts: fname "Weather file"; initbus "Create Simulink bus definition automatically"
      mask help:
      | Reads weather data from the specified binary file and outputs it as a Simulink bus signal.
      |
      | The utility function convertTMY3() to creates a .MAT file compatible with this block. Use of this block requires that a Simulink bus object named 'BusDef_Weather' be defined in the base workspace. See the block help for details.
      mask init:
      | % Run initialization callback
      | Weather_cb(gcb, 'init', fname, initbus);
      mask Help:
      | Import weather data from file
      | 
      | <h2>Description</h2>
      | This block reads weather data from a binary (.MAT) file and outputs it as a Simulink bus signal. Because the block uses Simulink's 'From File' block internally for file I/O, there are several requirements for it to function correctly; see Comments. The utility script <code>convertTMY3()</code> is available to convert TMY3-formatted weather data into a structure of MATLAB time series objects compatible with these requirements. See the <code>convertTMY3()</code> function documentation for details.
      | 
      | <h2>Output</h2>
      | Block output <b>data</b> is a Simulink bus containing weather data. The channels in the bus depend on the content of the weather file.
      | 
      | <h2>Parameters</h2>
      | The <b>weather file</b> parameter specifies the name of the weather file to load. This file must be in the MATLAB path.
      | 
      | If <b>Create Simulink bus definition automatically</b> is checked, then the block automatically creates the bus definition <code>BusDef_Weather</code> in the MATLAB workspace each time the block is initialized.
      | 
      | <h2>Comments</h2>
      | <ol>
      |   <li>The following requirements must be met for Simulink's <i>From File</i> block to function properly:
      |   <ol type="a">
      |     <li>The .MAT file of weather data must contain time series objects organized within a structure (struct) object called <code>ans</code>.</li>
      |     <li>The user must create a bus definition for the weather data named <code>BusDef_Weather</code> and save it to the base MATLAB workspace. (This bus definition will be automatically generated from the weather file if the <b>Create Simulink bus definition automatically</b> checkbox is checked.)</li>
      |     <li>The structure in the .MAT file must match the Simulink bus definition. (If the block is allowed to automatically generate the bus definition, this requirement will be satisfied.)</li>
      |     <li>The .MAT file must be version 7.3 or higher. Note that this is <i>not</i> the default .MAT file version for MATLAB R2013a.</li>
      |     <li>All time series in the .MAT file must have units of seconds; otherwise Simulink will interpret the time series incorrectly.</li>
      |    </ol>
      |    <li>If the .MAT file changes, the bus definition <code>BusDef_Weather</code> must be reinitialized.</li>
      |    <li>In some instances, Simulink will not reinitialize the <i>Weather Data</i> block when a model first loads, possibly leading to an error message that <code>BusDef_Weather</code> is missing. To force Simulink to reinitialize the block (and regenerate the bus definition), use the command
      |   <blockquote>
      |     <code>set_param(<i>blk</i>,'initbus',get_param(<i>blk</i>,'initbus'));</code>
      |   </blockquote>
      |   within the <i>PostLoadFcn</i> callback for the model, in which <code><i>blk</i></code> is the local path to the <i>Weather Data</i> block, for instance, <code>[gcs '/Weather Data']</code>.</li>
      | </ol>
      mask Display:
      | image(imread('SkyImage.png'))
      | port_label('output', 1, 'data');

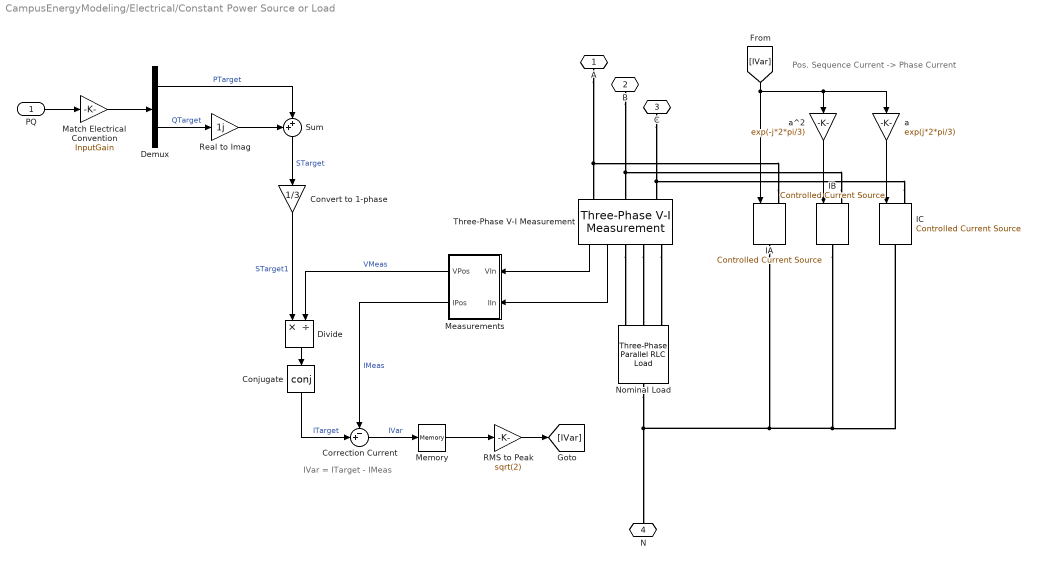
== system CampusEnergyModeling/Electrical/Constant Power Source or Load ==
  note: Pos. Sequence Current -> Phase Current
  note: IVar = ITarget - IMeas
  PQ : Inport  PortDimensions=2
  Conjugate : Math  Operator=conj  SaturateOnIntegerOverflow=on
  Convert to 1-phase : Gain  Gain=1/3
  Correction Current : Sum  Inputs=-+|
  Demux : Demux  Outputs=2
  Divide : Product  Inputs=*/
  IA : powerlib/Electrical Sources/Controlled Current Source  Initialize=off  Source_Type=AC  Amplitude=0  Phase=0  Frequency=0  Measurements=Current
  IB : powerlib/Electrical Sources/Controlled Current Source  Initialize=off  Source_Type=AC  Amplitude=0  Phase=0  Frequency=0  Measurements=Current
  IC : powerlib/Electrical Sources/Controlled Current Source  Initialize=off  Source_Type=AC  Amplitude=0  Phase=0  Frequency=0  Measurements=Current
  Match Electrical Convention : Gain  Gain=InputGain
  Measurements : Subsystem
  Memory : Memory
  Nominal Load : powerlib/Elements/Three-Phase Parallel RLC Load  LConnTagsString=A|B|C  RConnTagsString=N  Configuration=Y (neutral)  NominalVoltage=VNom  NominalFrequency=fNom  ActivePower=max(PNom*InputGain,1e-3)  InductivePower=max(QNom*InputGain,0)  CapacitivePower=max(-QNom*InputGain,0)  Measurements=None  LoadType=constant PQ
  RMS to Peak : Gain  Gain=sqrt(2)
  Real to Imag : Gain  Gain=1j
  Sum : Sum  Inputs=++|
  Three-Phase V-I Measurement : powerlib/Measurements/Three-Phase V-I Measurement  VoltageMeasurement=phase-to-ground  SetLabelV=off  LabelV=Vabc  Vpu=off  VpuLL=off  CurrentMeasurement=yes  SetLabelI=off  LabelI=Iabc  Ipu=off  Pbase=100e6  Vbase=VNom  OutputType=Complex  PhasorSimulation=on  PSBequivalent=0
  a : Gain  Gain=exp(j*2*pi/3)
  a^2 : Gain  Gain=exp(-j*2*pi/3)
  A : PMIOPort  Port=1  Side=Right
  B : PMIOPort  Port=2  Side=Right
  C : PMIOPort  Port=3  Side=Right
  N : PMIOPort  Port=4  Side=Right
  wires:
  Measurements/2(IPos) -> Correction Current/1  "IMeas"
  Measurements/1(VPos) -> Divide/2  "VMeas"
  Demux/1 -> Sum/2  "PTarget"
  Real to Imag/1 -> Sum/1
  Match Electrical Convention/1 -> Demux/1
  PQ/1 -> Match Electrical Convention/1
  Memory/1 -> RMS to Peak/1
  RMS to Peak/1 -> [IVar]
  Conjugate/1 -> Correction Current/2  "ITarget"
  Correction Current/1 -> Memory/1  "IVar"
  a/1 -> IC/1
  a^2/1 -> IB/1
  [IVar] -> a/1, a^2/1, IA/1
  Divide/1 -> Conjugate/1
  Convert to 1-phase/1 -> Divide/1  "STarget1"
  Sum/1 -> Convert to 1-phase/1  "STarget"
  Demux/2 -> Real to Imag/1  "QTarget"
  Three-Phase V-I Measurement/2 -> Measurements/2(IIn)
  Three-Phase V-I Measurement/1 -> Measurements/1(VIn)
  connections:
  IC/RConn1 -- N/RConn1 -- Nominal Load/RConn1 -- IA/RConn1 -- IB/RConn1
  Three-Phase V-I Measurement/RConn3 -- Nominal Load/LConn3
  Three-Phase V-I Measurement/RConn2 -- Nominal Load/LConn2
  Three-Phase V-I Measurement/RConn1 -- Nominal Load/LConn1
  IC/LConn1 -- Three-Phase V-I Measurement/LConn3 -- C/RConn1
  IB/LConn1 -- Three-Phase V-I Measurement/LConn2 -- B/RConn1
  IA/LConn1 -- Three-Phase V-I Measurement/LConn1 -- A/RConn1

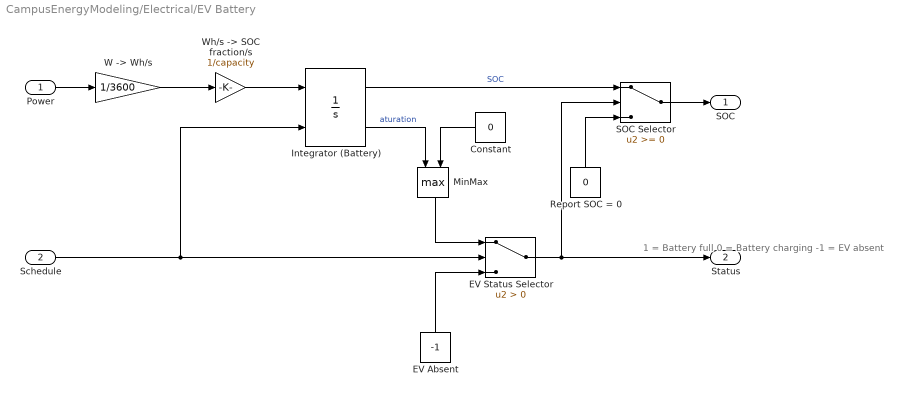
== system CampusEnergyModeling/Electrical/EV Battery ==
  note: 1 = Battery full
      | 0 = Battery charging
      | -1 = EV absent
  Power : Inport
  Schedule : Inport  Port=2
  Constant : Constant  Value=0
  EV Absent : Constant  Value=-1
  EV Status Selector : Switch  Criteria=u2 > Threshold
  Integrator (Battery) : Integrator  ExternalReset=rising  InitialCondition=initSOC  LimitOutput=on  UpperSaturationLimit=1  LowerSaturationLimit=0  ShowSaturationPort=on  ContinuousStateAttributes='SOC'
  MinMax : MinMax  Function=max  Inputs=2
  Report SOC = 0 : Constant  Value=0
  SOC Selector : Switch
  "W -> Wh/s" : Gain  Gain=1/3600
  "Wh/s -> SOC fraction/s" : Gain  Gain=1/capacity
  SOC : Outport
  Status : Outport  Port=2
  wires:
  "W -> Wh/s"/1 -> "Wh/s -> SOC fraction/s"/1
  Power/1 -> "W -> Wh/s"/1
  "Wh/s -> SOC fraction/s"/1 -> Integrator (Battery)/1
  Schedule/1 -> EV Status Selector/2, Integrator (Battery)/2
  EV Absent/1 -> EV Status Selector/3
  EV Status Selector/1 -> SOC Selector/2, Status/1
  Integrator (Battery)/2 -> MinMax/1  "aturation"
  MinMax/1 -> EV Status Selector/1
  Constant/1 -> MinMax/2
  Integrator (Battery)/1 -> SOC Selector/1  "SOC"
  SOC Selector/1 -> SOC/1
  Report SOC = 0/1 -> SOC Selector/3

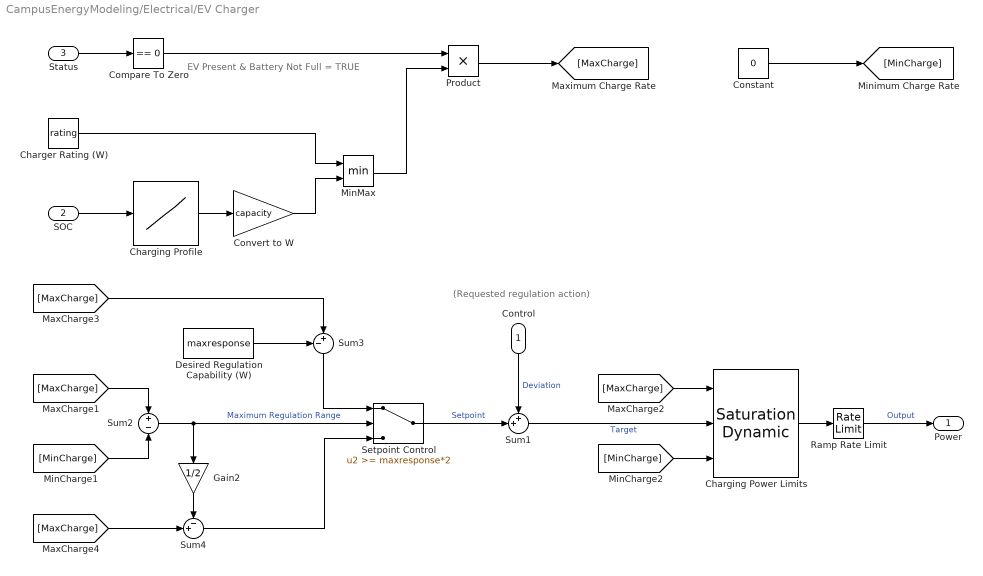
== system CampusEnergyModeling/Electrical/EV Charger ==
  note: EV Present & Battery Not Full = TRUE
  note: (Requested regulation action)
  Control : Inport
  SOC : Inport  Port=2
  Status : Inport  Port=3
  Charger Rating (W) : Constant  Value=rating
  Charging Power Limits : simulink/Discontinuities/Saturation Dynamic  OutMin=[]  OutMax=[]  OutDataTypeStr=Inherit: Same as second input  OutDataType=fixdt(1, 16)  OutScaling=2^-10  DoSatur=off
  Charging Profile : Lookup_n-D  NumberOfTableDimensions=1  BreakpointsForDimension1=[0.00 0.10 0.20 0.80 0.99 1.00]  IndexSearchMethod=Linear search  BeginIndexSearchUsingPreviousIndexResult=on  Table=[0.10 0.20 1.00 1.00 0.02 0.00]  ExtrapMethod=Clip  UseLastTableValue=on  RndMeth=Simplest  InputSameDT=on
  Compare To Zero : simulink/Logic and Bit Operations/Compare To Zero  relop===  OutDataTypeStr=boolean
  Constant : Constant  Value=0
  Convert to W : Gain  Gain=capacity
  Desired Regulation Capability (W) : Constant  Value=maxresponse
  Gain2 : Gain  Gain=1/2
  MinMax : MinMax  Inputs=2
  Product : Product
  Ramp Rate Limit : RateLimiter  RisingSlewLimit=ramp  FallingSlewLimit=-ramp  SampleTimeMode=inherited
  Setpoint Control : Switch  Threshold=maxresponse*2
  Sum1 : Sum  Inputs=++|
  Sum2 : Sum  Inputs=+-
  Sum3 : Sum  Inputs=-+|
  Sum4 : Sum  Inputs=-+|
  Power : Outport
  wires:
  Sum1/1 -> Charging Power Limits/2  "Target"
  Ramp Rate Limit/1 -> Power/1  "Output"
  SOC/1 -> Charging Profile/1
  Charging Profile/1 -> Convert to W/1
  Charging Power Limits/1 -> Ramp Rate Limit/1
  Status/1 -> Compare To Zero/1
  Compare To Zero/1 -> Product/1
  Convert to W/1 -> MinMax/2
  Charger Rating (W)/1 -> MinMax/1
  MinMax/1 -> Product/2
  Product/1 -> [MaxCharge]
  Constant/1 -> [MinCharge]
  Control/1 -> Sum1/1  "Deviation"
  [MaxCharge] -> Charging Power Limits/1
  [MinCharge] -> Charging Power Limits/3
  Sum2/1 -> Gain2/1, Setpoint Control/2  "Maximum Regulation Range"
  [MaxCharge] -> Sum2/1
  [MinCharge] -> Sum2/2
  Setpoint Control/1 -> Sum1/2  "Setpoint"
  Sum3/1 -> Setpoint Control/1
  [MaxCharge] -> Sum4/2
  Gain2/1 -> Sum4/1
  Sum4/1 -> Setpoint Control/3
  [MaxCharge] -> Sum3/2
  Desired Regulation Capability (W)/1 -> Sum3/1

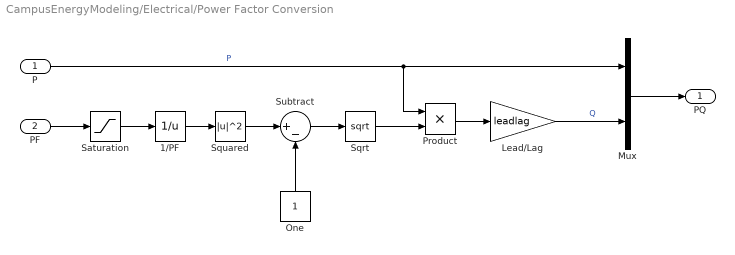
== system CampusEnergyModeling/Electrical/Power Factor Conversion ==
  P : Inport
  PF : Inport  Port=2
  1/PF : Math  Operator=reciprocal  SaturateOnIntegerOverflow=on
  Lead/Lag : Gain  Gain=leadlag
  Mux : Mux  Inputs=2
  One : Constant
  Product : Product
  Saturation : Saturate  UpperLimit=1  LowerLimit=0  ZeroCross=off
  Sqrt : Sqrt  SaturateOnIntegerOverflow=on
  Squared : Math  Operator=magnitude^2  SaturateOnIntegerOverflow=on
  Subtract : Sum  Inputs=|+-
  PQ : Outport
  wires:
  Subtract/1 -> Sqrt/1
  Sqrt/1 -> Product/2
  Mux/1 -> PQ/1
  Product/1 -> Lead/Lag/1
  PF/1 -> Saturation/1
  1/PF/1 -> Squared/1
  One/1 -> Subtract/2
  Squared/1 -> Subtract/1
  P/1 -> Product/1, Mux/1  "P"
  Lead/Lag/1 -> Mux/2  "Q"
  Saturation/1 -> 1/PF/1
